simulink model "KalmanTemperatureControl"  (R2020a)
settings: Solver=FixedStepAuto  StartTime=0.0  StopTime=10  RelTol=1e-3
settings Model: Creator=sadamu  LastModifiedBy=sadamu
settings SolverCC: AutoInsertRateTranBlk=on
settings DataIOCC: LimitDataPoints=on  SaveOutput=off  SignalLogging=off  DSMLogging=off  SaveTime=off
settings OptimizationCC: DefaultParameterBehavior=Inlined  DefaultUnderspecifiedDataType=single  OptimizeBlockIOStorage=off  BufferReuse=off  GlobalBufferReuse=off  ExpressionFolding=off  EnableMemcpy=off  PassReuseOutputArgsAs=Individual arguments  LocalBlockOutputs=off  ZeroExternalMemoryAtStartup=off  ZeroInternalMemoryAtStartup=off  NoFixptDivByZeroProtection=on  OptimizeDataStoreBuffers=off  BusAssignmentInplaceUpdate=off  OptimizationLevel=level0  OptimizationPriority=Speed  MultiThreadedLoops=on  EfficientTunableParamExpr=on
settings DebuggingCC: AlgebraicLoopMsg=error  SingleTaskRateTransMsg=error  ParameterTunabilityLossMsg=error  AllowSymbolicDim=off  SFUnexpectedBacktrackingDiag=warning  SFNoUnconditionalDefaultTransitionDiag=warning  SFExecutionAtInitializationDiag=none  ArithmeticOperatorsInVariantConditions=warning
settings SFSimCC: SimUseLocalCustomCode=off  MATLABDynamicMemAlloc=off  CustomCodeUndefinedFunction=UseInterfaceOnly
settings RTWCC: SystemTargetFile=ert.tlc  GenCodeOnly=on  TemplateMakefile=ert_default_tmf  GenerateReport=on  RTWUseLocalCustomCode=off  BuildConfiguration=Debug  LaunchReport=on
settings CodeAppCC: GenerateComments=off  IgnoreCustomStorageClasses=off  OperatorAnnotations=on  SimulinkDataObjDesc=on  SFDataObjDesc=on  InsertBlockDesc=on  EnableCustomComments=on
settings ERTTargetCC: GenerateSampleERTMain=on  SuppressErrorStatus=on  InlinedParameterPlacement=NonHierarchical  ERTCustomFileTemplate=example_file_process.tlc

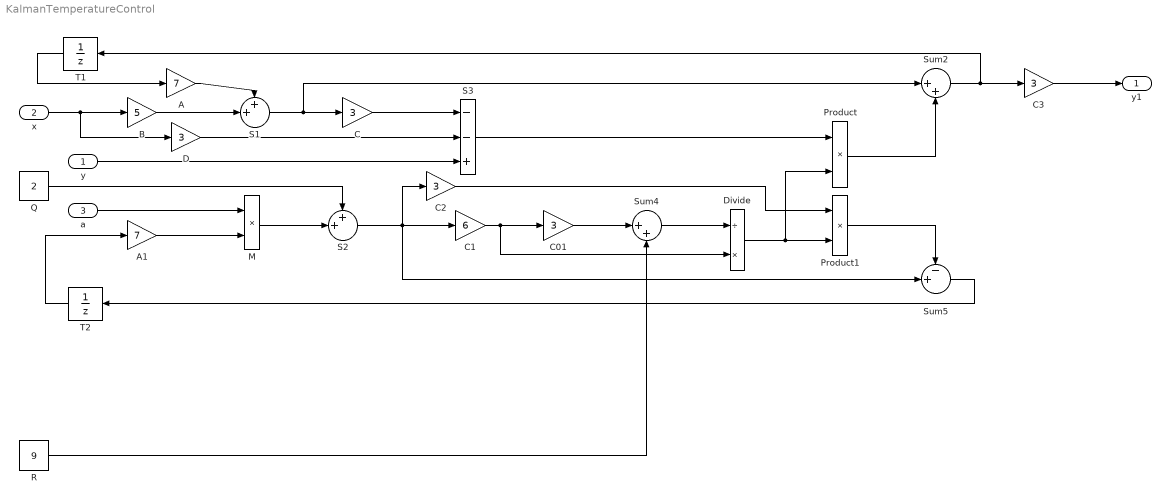
== system KalmanTemperatureControl ==
  y : Inport
  x : Inport  Port=2
  a : Inport  Port=3
  A : Gain  Gain=7  OutDataTypeStr=int32  RndMeth=Simplest
  A1 : Gain  Gain=7  OutDataTypeStr=int32
  B : Gain  Gain=5  OutDataTypeStr=int32  RndMeth=Simplest
  C : Gain  Gain=3  OutDataTypeStr=int32  RndMeth=Simplest
  C01 : Gain  Gain=3  OutDataTypeStr=int32
  C1 : Gain  Gain=6  OutDataTypeStr=int32  RndMeth=Simplest
  C2 : Gain  Gain=3  OutDataTypeStr=int32  RndMeth=Simplest
  C3 : Gain  Gain=3  OutDataTypeStr=int32  RndMeth=Simplest
  D : Gain  Gain=3  OutDataTypeStr=int32  RndMeth=Simplest
  Divide : Product  Inputs=/*  OutDataTypeStr=int32  RndMeth=Zero
  M : Product  OutDataTypeStr=int32
  Product : Product  OutDataTypeStr=int32
  Product1 : Product  OutDataTypeStr=int32
  Q : Constant  Value=2  OutDataTypeStr=int32
  R : Constant  Value=9  OutDataTypeStr=int32
  S1 : Sum  Inputs=++|  OutDataTypeStr=int32
  S2 : Sum  Inputs=++|
  S3 : Sum  Inputs=--+  OutDataTypeStr=int32  RndMeth=Simplest
  Sum2 : Sum  Inputs=|++  OutDataTypeStr=int32
  Sum4 : Sum  Inputs=|++  OutDataTypeStr=int32  RndMeth=Simplest
  Sum5 : Sum  Inputs=-+|  OutDataTypeStr=int32
  T1 : UnitDelay  SampleTime=-1
  T2 : UnitDelay  SampleTime=-1
  y1 : Outport
  wires:
  M/1 -> S2/2
  S2/1 -> Sum5/2, C2/1, C1/1
  S1/1 -> C/1, Sum2/1
  Sum2/1 -> C3/1, T1/1
  Product/1 -> Sum2/2
  Q/1 -> S2/1
  C01/1 -> Sum4/1
  S3/1 -> Product/1
  C2/1 -> Product1/1
  x/1 -> D/1, B/1
  T2/1 -> A1/1
  R/1 -> Sum4/2
  Product1/1 -> Sum5/1
  Sum4/1 -> Divide/1
  a/1 -> M/1
  C1/1 -> C01/1, Divide/2
  C3/1 -> y1/1
  D/1 -> S3/2
  Divide/1 -> Product/2, Product1/2
  Sum5/1 -> T2/1
  T1/1 -> A/1
  C/1 -> S3/1
  B/1 -> S1/2
  A1/1 -> M/2
  y/1 -> S3/3
  A/1 -> S1/1
